simulink model "osqp_test"  (R2018b)
settings: Solver=FixedStepAuto  StartTime=0.0  StopTime=10.0  FixedStep=0.1  RelTol=1e-3
undefined symbols (not defined in the file): A_x_par, l_par, P_x_par, q_par, u_par
settings Model: Creator=salih  LastModifiedBy=ge34qer
settings OptimizationCC: DefaultParameterBehavior=Inlined  EnhancedBackFolding=on  PassReuseOutputArgsAs=Individual arguments  OptimizeBlockOrder=speed  DifferentSizesBufferReuse=on  OptimizationCustomize=off
settings DebuggingCC: ParameterTunabilityLossMsg=error
settings SFSimCC: MATLABDynamicMemAlloc=off
settings RTWCC: SystemTargetFile=ert.tlc  TemplateMakefile=ert_default_tmf  GenerateReport=on  CustomSource=osqp_wrapper.c  CustomLibrary=lib/libosqp_mingw.lib  IncludeHyperlinkInReport=on  LaunchReport=on  TargetLang=C++  GenerateTraceInfo=on  GenerateTraceReport=on  GenerateTraceReportSl=on  GenerateTraceReportSf=on  GenerateTraceReportEml=on
settings CodeAppCC: ForceParamTrailComments=on  IgnoreCustomStorageClasses=off  OperatorAnnotations=on  SimulinkDataObjDesc=on  SFDataObjDesc=on  InsertBlockDesc=on
settings ERTTargetCC: TargetLangStandard=C++03 (ISO)  GenerateSampleERTMain=on  MatFileLogging=on  MultiInstanceERTCode=on  CodeInterfacePackaging=Reusable function  InlinedParameterPlacement=NonHierarchical  MultiInstanceErrorCode=None  RootIOFormat=Structure reference  ERTCustomFileTemplate=example_file_process.tlc

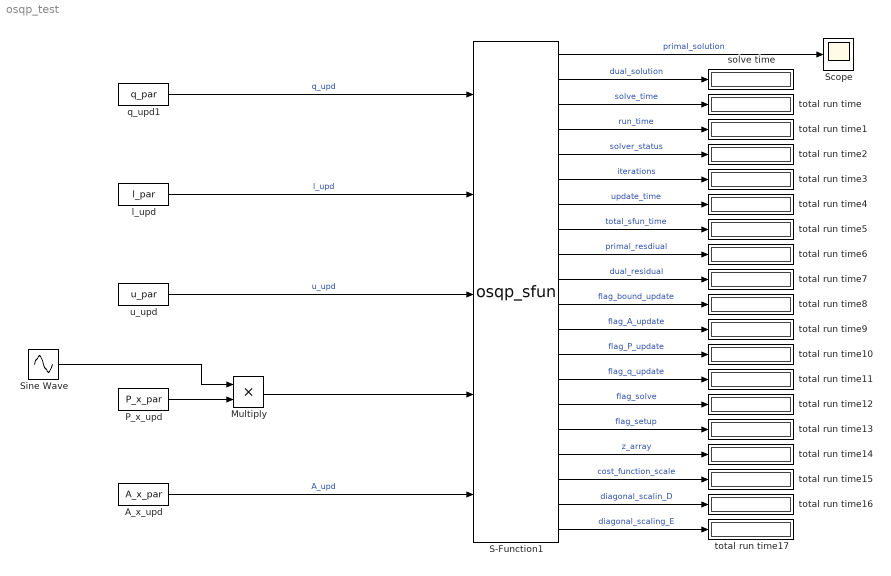
== system osqp_test ==
  "A_x_upd " : Constant  Value=A_x_par
  Multiply : Product
  "P_x_upd " : Constant  Value=P_x_par
  S-Function1 : S-Function  FunctionName=osqp_sfun  Parameters=q_par, m, n, P_x_par, P_i_par, P_p_par, A_x_par, A_i_par, A_p_par, l_par, u_par, trigger_print, trigger_Pupdate  SFunctionDeploymentMode=off  EnableBusSupport=off
  Scope : Scope
  Sine Wave : Sin  Amplitude=0.1  Bias=2  SampleTime=0.1
  l_upd : Constant  Value=l_par
  q_upd1 : Constant  Value=q_par
  solve time : Display
  total run time{,1..17} (18 alike) : Display
  u_upd : Constant  Value=u_par
  wires:
  S-Function1/1 -> Scope/1  "primal_solution"
  l_upd/1 -> S-Function1/2  "l_upd"
  u_upd/1 -> S-Function1/3  "u_upd"
  S-Function1/2 -> solve time/1  "dual_solution"
  S-Function1/3 -> total run time/1  "solve_time"
  S-Function1/5 -> total run time2/1  "solver_status"
  q_upd1/1 -> S-Function1/1  "q_upd"
  S-Function1/6 -> total run time3/1  "iterations"
  "A_x_upd "/1 -> S-Function1/5  "A_upd"
  S-Function1/4 -> total run time1/1  "run_time"
  S-Function1/7 -> total run time4/1  "update_time"
  S-Function1/8 -> total run time5/1  "total_sfun_time"
  S-Function1/9 -> total run time6/1  "primal_resdiual"
  S-Function1/10 -> total run time7/1  "dual_residual"
  S-Function1/11 -> total run time8/1  "flag_bound_update"
  S-Function1/12 -> total run time9/1  "flag_A_update"
  S-Function1/13 -> total run time10/1  "flag_P_update"
  "P_x_upd "/1 -> Multiply/2
  Sine Wave/1 -> Multiply/1
  Multiply/1 -> S-Function1/4
  S-Function1/14 -> total run time11/1  "flag_q_update"
  S-Function1/15 -> total run time12/1  "flag_solve"
  S-Function1/16 -> total run time13/1  "flag_setup"
  S-Function1/17 -> total run time14/1  "z_array"
  S-Function1/18 -> total run time15/1  "cost_function_scale"
  S-Function1/19 -> total run time16/1  "diagonal_scalin_D"
  S-Function1/20 -> total run time17/1  "diagonal_scaling_E"
